simulink model "trackerSys"  (R2014b)
settings: Solver=ode45  StartTime=0.0  StopTime=10  RelTol=1e-3
values from neighbouring files (symbols this model uses):
  A = [1 0 dt 0; 0 1 0 dt; 0 0 1 0; 0 0 0 1]    [Part3.m]
  B = [(dt^2/2); (dt^2/2); dt; dt]    [Part3.m]
  C = [1 0 0 0; 0 1 0 0]    [Part3.m]
  F = -F    [Part3.m]
  H = -H'    [Part3.m]
  M = -inv(C*inv(A+B*F)*B)    [Part3.m]
  x0_o = [0.5 0.5]'    [Part3.m]
undefined symbols (not defined in the file or in its folder): D
settings Model: CovSFcnEnable=on  Creator=Benny  LastModifiedBy=123
settings OptimizationCC: UseDivisionForNetSlopeComputation=off  SimCompilerOptimization=off
settings DebuggingCC: SolverPrmCheckMsg=none  FrameProcessingCompatibilityMsg=error
settings RTWCC: RTWCompilerOptimization=off

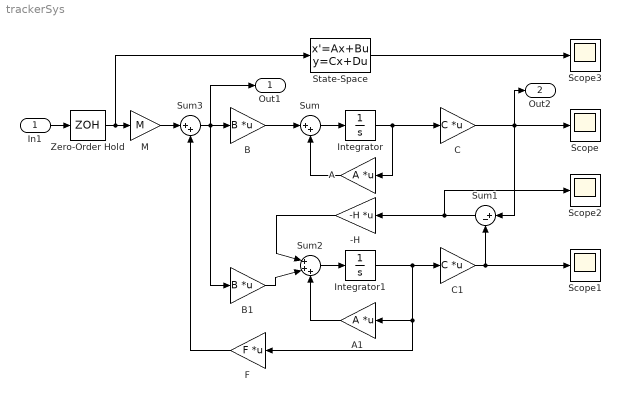
== system trackerSys ==
  In1 : Inport
  -H : Gain  Gain=-H  Multiplication=Matrix(K*u)
  A : Gain  Gain=A  Multiplication=Matrix(K*u)
  A1 : Gain  Gain=A  Multiplication=Matrix(K*u)
  B : Gain  Gain=B  Multiplication=Matrix(K*u)
  B1 : Gain  Gain=B  Multiplication=Matrix(K*u)
  C : Gain  Gain=C  Multiplication=Matrix(K*u)
  C1 : Gain  Gain=C  Multiplication=Matrix(K*u)
  F : Gain  Gain=F  Multiplication=Matrix(K*u)
  Integrator : Integrator
  Integrator1 : Integrator  InitialCondition=x0_o
  M : Gain  Gain=M
  Scope{,1..3} (4 alike) : Scope
      Scope2 settings: SaveName=ScopeData2
      Scope3 settings: SaveName=ScopeData3
  State-Space : StateSpace  A=A  B=B  C=C  D=D  X0=0
  Sum : Sum  Inputs=|++
  Sum1 : Sum  Inputs=|+-
  Sum2 : Sum  Inputs=|+++
  Sum3 : Sum  Inputs=|++
  Zero-Order Hold : ZeroOrderHold
  Out1 : Outport
  Out2 : Outport  Port=2
  wires:
  In1/1 -> Zero-Order Hold/1
  B/1 -> Sum/1
  Sum/1 -> Integrator/1
  A/1 -> Sum/2
  Integrator/1 -> C/1, A/1
  C/1 -> Out2/1, Sum1/1, Scope/1
  Sum1/1 -> Scope2/1, -H/1
  C1/1 -> Sum1/2, Scope1/1
  Integrator1/1 -> F/1, A1/1, C1/1
  -H/1 -> Sum2/1
  Sum2/1 -> Integrator1/1
  A1/1 -> Sum2/3
  B1/1 -> Sum2/2
  M/1 -> Sum3/1
  Sum3/1 -> Out1/1, B1/1, B/1
  F/1 -> Sum3/2
  State-Space/1 -> Scope3/1
  Zero-Order Hold/1 -> State-Space/1, M/1
